simulink model "splits_m"  (Simulink 8.5)
settings: Solver=ode45  SolverMode=SingleTasking  StartTime=0.0  StopTime=999999  MaxStep=10  RelTol=1e-3  AbsTol=1e-3
values from neighbouring files (symbols this model uses):
  U = st_Varia('LongNames')    [splits_i.m]
  x0 = []    [splits_i.m]    (also in splits_s.m = x0)
undefined symbols (not defined in the file or in its folder): B
settings Model: Creator=M.Sparnaaij  LastModifiedBy=Martijn
settings DataIOCC: LimitDataPoints=off  SaveOutput=off  SaveTime=off  SignalLoggingName=sigsOut
settings OptimizationCC: BooleanDataType=off
settings DebuggingCC: SaveWithParameterizedLinksMsg=none  SignalResolutionControl=TryResolveAllWithWarning  MultiTaskDSMMsg=warning  MultiTaskCondExecSysMsg=none  FcnCallInpInsideContextMsg=EnableAllAsWarning  StrictBusMsg=None
settings HardwareCC: TargetUnknown=on

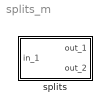
== system splits_m ==
  splits : Subsystem  Description=splits
      mask init:
      | filenaam='.\StimelaData\splits_p.mat';
      | 
      | [Pn,Fn,Fext]=Fileprop(filenaam);
      | 
      | errstr = st_UniqName(filenaam,'filenaam=''','SubSystem','OpenFcn');
      | if errstr, error([errstr 'The filename "' filenaam '" is already in use. Choose a different filename.']), end
      | 
      | P = splits_p(filenaam);
      | [B,x0,U]=splits_i(filenaam);
      settings: OpenFcn=|
      | filenaam='.\StimelaData\splits_p.mat';
      | st_ParameterInput('init',gcb,filenaam,'splits');
      mask Display:
      | plot(0,0,100,100,[0 20],[50 50],[0 20],[55 55],[80 100],[80 80],[80 100],[85 85],[80 100],[ 20 20],[80 100],[ 15 15],[20 80 80 20 20],[10 10 90  90 10]);
      | disp('')
      | text(50,50,'splits', 'horizontalAlignment', 'center', 'verticalAlignment', 'middle');
      | text(50,0,Fn, 'horizontalAlignment', 'center', 'verticalAlignment', 'base');

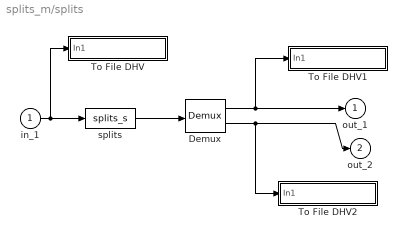
== system splits_m/splits ==
  in_1 : Inport
  Demux : Demux  Outputs=[U.Number B.Measurements]
  To File DHV : Subsystem  mask(To File DHV){naam=[filenaam(1:length(filenaam)-4) '_in.sti']}
      mask prompts: naam "Naam van bestand"
      mask init:
      | set_param([gcb '/To File'],'Filename',naam);
      mask Display: disp(naam)
  To File DHV1 : Subsystem  mask(To File DHV){naam=[filenaam(1:length(filenaam)-4) '_out.sti']}
      mask prompts: naam "Naam van bestand"
      mask init:
      | set_param([gcb '/To File'],'Filename',naam);
      mask Display: disp(naam)
  To File DHV2 : Subsystem  mask(To File DHV){naam=[filenaam(1:length(filenaam)-4) '_EM.sti']}
      mask prompts: naam "Naam van bestand"
      mask init:
      | set_param([gcb '/To File'],'Filename',naam);
      mask Display: disp(naam)
  splits : S-Function  FunctionName=splits_s  Parameters=B,x0,U,P
  out_1 : Outport  InitialOutput=0
  out_2 : Outport  Port=2  InitialOutput=0
  wires:
  in_1/1 -> To File DHV/1(In1), splits/1
  Demux/2 -> To File DHV2/1(In1), out_2/1
  Demux/1 -> To File DHV1/1(In1), out_1/1
  splits/1 -> Demux/1

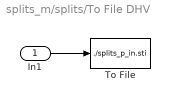
== system splits_m/splits/To File DHV ==
  In1 : Inport
  To File : ToFile  Filename=./splits_p_in.sti  MatrixName=splitsin
  wires:
  In1/1 -> To File/1

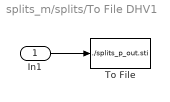
== system splits_m/splits/To File DHV1 ==
  In1 : Inport
  To File : ToFile  Filename=./splits_p_out.sti  MatrixName=splitsout
  wires:
  In1/1 -> To File/1

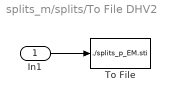
== system splits_m/splits/To File DHV2 ==
  In1 : Inport
  To File : ToFile  Filename=./splits_p_EM.sti  MatrixName=splitsEM
  wires:
  In1/1 -> To File/1
